simulink model "automata_learning"  (R2022a)
settings: Solver=FixedStepAuto  StartTime=0.0  StopTime=10.0  FixedStep=0.01  RelTol=1e-3
settings Model: Creator=diego  LastModifiedBy=diego

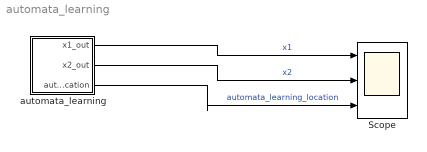
== system automata_learning ==
  Scope : Scope  NumInputPorts=3
  automata_learning : Stateflow chart  TreatAsAtomicUnit=on
  wires:
  automata_learning/1(x1_out) -> Scope/1  "x1"
  automata_learning/2(x2_out) -> Scope/2  "x2"
  automata_learning/3(automata_learning_location) -> Scope/3  "automata_learning_location"

== stateflow chart automata_learning/automata_learning ==
  settings: updateMethod=CONTINUOUS
  state loc1
    du:
    x1_dot = 0.153649240732193 * (exp(0.62066251039505 * x1 + 0.017139941453933716 * x2 + 0.2983952462673187) - 1.0) / (exp(0.62066251039505 * x1 + 0.017139941453933716 * x2 + 0.2983952462673187) + 1.0) - 0.2748902142047882 * (exp(0.430800199508667 * x1 + 0.22947368025779724 * x2 - 0.22418212890625) - 1.0) / (exp(0.430800199508667 * x1 + 0.22947368025779724 * x2 - 0.22418212890625) + 1.0) + 0.32443326711654663 * (exp(0.6266034245491028 * x2 - 0.5493556261062622 * x1 + 0.17436186969280243) - 1.0) / (exp(0.6266034245491028 * x2 - 0.5493556261062622 * x1 + 0.17436186969280243) + 1.0) + 0.3301161229610443 * (exp(0.6688907146453857 * x1 + 0.6354950666427612 * x2 + 0.28973063826560974) - 1.0) / (exp(0.6688907146453857 * x1 + 0.6354950666427612 * x2 + 0.28973063826560974) + 1.0) + 0.3717308044433594 * (exp(0.5966212749481201 * x1 - 0.30495092272758484 * x2 + 0.17112641036510468) - 1.0) / (exp(0.5966212749481201 * x1 - 0.30495092272758484 * x2 + 0.17112641036510468) + 1.0) + 0.15974511206150055 * (exp(0.5138949155807495 * x2 - 0.872249186038971 * x1 + 0.12989071011543274) - 1.0) / (exp(0.5138949155807495 * x2 - 0.872249186038971 * x1 + 0.12989071011543274) + 1.0) + 0.09516903012990952 * (exp(0.5174744129180908 * x1 - 0.458869606256485 * x2 + 0.07007770240306854) - 1.0) / (exp(0.5174744129180908 * x1 - 0.458869606256485 * x2 + 0.07007770240306854) + 1.0) + 0.13788394629955292 * (exp(0.3413529098033905 * x1 - 0.13695278763771057 * x2 + 0.0960288867354393) - 1.0) / (exp(0.3413529098033905 * x1 - 0.13695278763771057 * x2 + 0.0960288867354393) + 1.0) + 0.23488743603229523 * (exp(0.459713339805603 * x1 + 0.2586129903793335 * x2 + 0.14161019027233124) - 1.0) / (exp(0.459713339805603 * x1 + 0.2586129903793335 * x2 + 0.14161019027233124) + 1.0) - 0.38932523131370544 * (exp(0.16752173006534576 * x1 + 0.30755898356437683 * x2 - 0.18332701921463013) - 1.0) / (exp(0.16752173006534576 * x1 + 0.30755898356437683 * x2 - 0.18332701921463013) + 1.0) + 0.4114132523536682 * (exp(0.4421512186527252 * x2 - 0.0019959965720772743 * x1 + 0.1608879119157791) - 1.0) / (exp(0.4421512186527252 * x2 - 0.0019959965720772743 * x1 + 0.1608879119157791) + 1.0) + 0.2618536949157715 * (exp(0.7581536173820496 * x2 - 0.5491491556167603 * x1 + 0.1869184970855713) - 1.0) / (exp(0.7581536173820496 * x2 - 0.5491491556167603 * x1 + 0.1869184970855713) + 1.0) - 0.28562095761299133 * (exp(0.5797051787376404 * x1 + 0.4280661344528198 * x2 - 0.32014745473861694) - 1.0) / (exp(0.5797051787376404 * x1 + 0.4280661344528198 * x2 - 0.32014745473861694) + 1.0) - 0.022995460778474808 * (exp(0.5465248227119446 * x1 - 0.7955937385559082 * x2 + 0.025239817798137665) - 1.0) / (exp(0.5465248227119446 * x1 - 0.7955937385559082 * x2 + 0.025239817798137665) + 1.0) + 0.40521523356437683 * (exp(0.015660669654607773 * x1 - 0.0256962887942791 * x2 + 0.21741506457328796) - 1.0) / (exp(0.015660669654607773 * x1 - 0.0256962887942791 * x2 + 0.21741506457328796) + 1.0) + 0.35603979229927063 * (exp(0.20083804428577423 * x1 - 0.17433811724185944 * x2 + 0.1748630851507187) - 1.0) / (exp(0.20083804428577423 * x1 - 0.17433811724185944 * x2 + 0.1748630851507187) + 1.0) + 0.36211273074150085 * (exp(0.09791313111782074 * x1 + 0.12835988402366638 * x2 + 0.23166249692440033) - 1.0) / (exp(0.09791313111782074 * x1 + 0.12835988402366638 * x2 + 0.23166249692440033) + 1.0) + 0.05281674489378929 * (exp(0.6614029407501221 * x1 - 0.7321106195449829 * x2 + 0.10560699552297592) - 1.0) / (exp(0.6614029407501221 * x1 - 0.7321106195449829 * x2 + 0.10560699552297592) + 1.0) + 0.2983291745185852 * (exp(0.6240413188934326 * x2 - 0.6195738315582275 * x1 + 0.24919748306274414) - 1.0) / (exp(0.6240413188934326 * x2 - 0.6195738315582275 * x1 + 0.24919748306274414) + 1.0) - 0.07643954455852509 * (exp(0.37432658672332764 * x1 + 0.13084420561790466 * x2 - 0.061473298817873) - 1.0) / (exp(0.37432658672332764 * x1 + 0.13084420561790466 * x2 - 0.061473298817873) + 1.0) + 0.07931482791900635 * (exp(0.6290643215179443 * x1 + 0.7032239437103271 * x2 + 0.029886124655604362) - 1.0) / (exp(0.6290643215179443 * x1 + 0.7032239437103271 * x2 + 0.029886124655604362) + 1.0) + 0.3452206552028656 * (exp(0.46229633688926697 * x1 - 0.17825168371200562 * x2 + 0.33221080899238586) - 1.0) / (exp(0.46229633688926697 * x1 - 0.17825168371200562 * x2 + 0.33221080899238586) + 1.0) - 0.3357248306274414 * (exp(0.32255837321281433 * x1 + 0.4906807243824005 * x2 - 0.171269491314888) - 1.0) / (exp(0.32255837321281433 * x1 + 0.4906807243824005 * x2 - 0.171269491314888) + 1.0) + 0.032010987401008606 * (exp(0.49095281958580017 * x1 - 0.07064257562160492 * x2 + 0.20939995348453522) - 1.0) / (exp(0.49095281958580017 * x1 - 0.07064257562160492 * x2 + 0.20939995348453522) + 1.0) + 0.26413223147392273 * (exp(0.45438820123672485 * x1 - 0.2572150230407715 * x2 + 0.24137400090694427) - 1.0) / (exp(0.45438820123672485 * x1 - 0.2572150230407715 * x2 + 0.24137400090694427) + 1.0) - 0.3747853934764862 * (exp(0.8867902755737305 * x1 + 0.4323332607746124 * x2 - 0.3189244270324707) - 1.0) / (exp(0.8867902755737305 * x1 + 0.4323332607746124 * x2 - 0.3189244270324707) + 1.0) + 0.41086137294769287 * (exp(0.36686065793037415 * x2 - 0.000020963780116289854 * x1 + 0.24850977957248688) - 1.0) / (exp(0.36686065793037415 * x2 - 0.000020963780116289854 * x1 + 0.24850977957248688) + 1.0) + 0.5473085641860962 * (exp(0.20481422543525696 * x1 - 0.47845104336738586 * x2 + 0.3234947621822357) - 1.0) / (exp(0.20481422543525696 * x1 - 0.47845104336738586 * x2 + 0.3234947621822357) + 1.0) + 0.05670561641454697 * (exp(0.34265992045402527 * x1 + 0.7918558120727539 * x2 + 0.11939319968223572) - 1.0) / (exp(0.34265992045402527 * x1 + 0.7918558120727539 * x2 + 0.11939319968223572) + 1.0) + 0.39071744680404663 * (exp(0.49077701568603516 * x1 - 0.11882556974887848 * x2 + 0.2540743947029114) - 1.0) / (exp(0.49077701568603516 * x1 - 0.11882556974887848 * x2 + 0.2540743947029114) + 1.0) + 0.13067974150180817;
    x2_dot = 0.4149567782878876 * (exp(0.430800199508667 * x1 + 0.22947368025779724 * x2 - 0.22418212890625) - 1.0) / (exp(0.430800199508667 * x1 + 0.22947368025779724 * x2 - 0.22418212890625) + 1.0) + 0.033265016973018646 * (exp(0.62066251039505 * x1 + 0.017139941453933716 * x2 + 0.2983952462673187) - 1.0) / (exp(0.62066251039505 * x1 + 0.017139941453933716 * x2 + 0.2983952462673187) + 1.0) + 0.11906763911247253 * (exp(0.6266034245491028 * x2 - 0.5493556261062622 * x1 + 0.17436186969280243) - 1.0) / (exp(0.6266034245491028 * x2 - 0.5493556261062622 * x1 + 0.17436186969280243) + 1.0) + 0.09495125710964203 * (exp(0.6688907146453857 * x1 + 0.6354950666427612 * x2 + 0.28973063826560974) - 1.0) / (exp(0.6688907146453857 * x1 + 0.6354950666427612 * x2 + 0.28973063826560974) + 1.0) + 0.4443686902523041 * (exp(0.5966212749481201 * x1 - 0.30495092272758484 * x2 + 0.17112641036510468) - 1.0) / (exp(0.5966212749481201 * x1 - 0.30495092272758484 * x2 + 0.17112641036510468) + 1.0) - 0.4195578992366791 * (exp(0.5138949155807495 * x2 - 0.872249186038971 * x1 + 0.12989071011543274) - 1.0) / (exp(0.5138949155807495 * x2 - 0.872249186038971 * x1 + 0.12989071011543274) + 1.0) + 0.46499332785606384 * (exp(0.5174744129180908 * x1 - 0.458869606256485 * x2 + 0.07007770240306854) - 1.0) / (exp(0.5174744129180908 * x1 - 0.458869606256485 * x2 + 0.07007770240306854) + 1.0) + 0.3947281837463379 * (exp(0.3413529098033905 * x1 - 0.13695278763771057 * x2 + 0.0960288867354393) - 1.0) / (exp(0.3413529098033905 * x1 - 0.13695278763771057 * x2 + 0.0960288867354393) + 1.0) + 0.36730241775512695 * (exp(0.459713339805603 * x1 + 0.2586129903793335 * x2 + 0.14161019027233124) - 1.0) / (exp(0.459713339805603 * x1 + 0.2586129903793335 * x2 + 0.14161019027233124) + 1.0) - 0.266009658575058 * (exp(0.16752173006534576 * x1 + 0.30755898356437683 * x2 - 0.18332701921463013) - 1.0) / (exp(0.16752173006534576 * x1 + 0.30755898356437683 * x2 - 0.18332701921463013) + 1.0) + 0.4192095696926117 * (exp(0.4421512186527252 * x2 - 0.0019959965720772743 * x1 + 0.1608879119157791) - 1.0) / (exp(0.4421512186527252 * x2 - 0.0019959965720772743 * x1 + 0.1608879119157791) + 1.0) + 0.008743703365325928 * (exp(0.7581536173820496 * x2 - 0.5491491556167603 * x1 + 0.1869184970855713) - 1.0) / (exp(0.7581536173820496 * x2 - 0.5491491556167603 * x1 + 0.1869184970855713) + 1.0) + 0.14651131629943848 * (exp(0.5797051787376404 * x1 + 0.4280661344528198 * x2 - 0.32014745473861694) - 1.0) / (exp(0.5797051787376404 * x1 + 0.4280661344528198 * x2 - 0.32014745473861694) + 1.0) - 0.3324713110923767 * (exp(0.5465248227119446 * x1 - 0.7955937385559082 * x2 + 0.025239817798137665) - 1.0) / (exp(0.5465248227119446 * x1 - 0.7955937385559082 * x2 + 0.025239817798137665) + 1.0) + 0.1831395924091339 * (exp(0.015660669654607773 * x1 - 0.0256962887942791 * x2 + 0.21741506457328796) - 1.0) / (exp(0.015660669654607773 * x1 - 0.0256962887942791 * x2 + 0.21741506457328796) + 1.0) + 0.3701251149177551 * (exp(0.20083804428577423 * x1 - 0.17433811724185944 * x2 + 0.1748630851507187) - 1.0) / (exp(0.20083804428577423 * x1 - 0.17433811724185944 * x2 + 0.1748630851507187) + 1.0) + 0.1405045986175537 * (exp(0.09791313111782074 * x1 + 0.12835988402366638 * x2 + 0.23166249692440033) - 1.0) / (exp(0.09791313111782074 * x1 + 0.12835988402366638 * x2 + 0.23166249692440033) + 1.0) - 0.22994273900985718 * (exp(0.6614029407501221 * x1 - 0.7321106195449829 * x2 + 0.10560699552297592) - 1.0) / (exp(0.6614029407501221 * x1 - 0.7321106195449829 * x2 + 0.10560699552297592) + 1.0) - 0.3847588896751404 * (exp(0.6240413188934326 * x2 - 0.6195738315582275 * x1 + 0.24919748306274414) - 1.0) / (exp(0.6240413188934326 * x2 - 0.6195738315582275 * x1 + 0.24919748306274414) + 1.0) + 0.43302276730537415 * (exp(0.37432658672332764 * x1 + 0.13084420561790466 * x2 - 0.061473298817873) - 1.0) / (exp(0.37432658672332764 * x1 + 0.13084420561790466 * x2 - 0.061473298817873) + 1.0) + 0.3945055603981018 * (exp(0.6290643215179443 * x1 + 0.7032239437103271 * x2 + 0.029886124655604362) - 1.0) / (exp(0.6290643215179443 * x1 + 0.7032239437103271 * x2 + 0.029886124655604362) + 1.0) - 0.23404325544834137 * (exp(0.46229633688926697 * x1 - 0.17825168371200562 * x2 + 0.33221080899238586) - 1.0) / (exp(0.46229633688926697 * x1 - 0.17825168371200562 * x2 + 0.33221080899238586) + 1.0) - 0.26820316910743713 * (exp(0.32255837321281433 * x1 + 0.4906807243824005 * x2 - 0.171269491314888) - 1.0) / (exp(0.32255837321281433 * x1 + 0.4906807243824005 * x2 - 0.171269491314888) + 1.0) + 0.058586183935403824 * (exp(0.49095281958580017 * x1 - 0.07064257562160492 * x2 + 0.20939995348453522) - 1.0) / (exp(0.49095281958580017 * x1 - 0.07064257562160492 * x2 + 0.20939995348453522) + 1.0) + 0.1390489935874939 * (exp(0.45438820123672485 * x1 - 0.2572150230407715 * x2 + 0.24137400090694427) - 1.0) / (exp(0.45438820123672485 * x1 - 0.2572150230407715 * x2 + 0.24137400090694427) + 1.0) + 0.4438546895980835 * (exp(0.8867902755737305 * x1 + 0.4323332607746124 * x2 - 0.3189244270324707) - 1.0) / (exp(0.8867902755737305 * x1 + 0.4323332607746124 * x2 - 0.3189244270324707) + 1.0) + 0.0753171443939209 * (exp(0.36686065793037415 * x2 - 0.000020963780116289854 * x1 + 0.24850977957248688) - 1.0) / (exp(0.36686065793037415 * x2 - 0.000020963780116289854 * x1 + 0.24850977957248688) + 1.0) - 0.1991405040025711 * (exp(0.20481422543525696 * x1 - 0.47845104336738586 * x2 + 0.3234947621822357) - 1.0) / (exp(0.20481422543525696 * x1 - 0.47845104336738586 * x2 + 0.3234947621822357) + 1.0) - 0.3242756724357605 * (exp(0.34265992045402527 * x1 + 0.7918558120727539 * x2 + 0.11939319968223572) - 1.0) / (exp(0.34265992045402527 * x1 + 0.7918558120727539 * x2 + 0.11939319968223572) + 1.0) + 0.1375180333852768 * (exp(0.49077701568603516 * x1 - 0.11882556974887848 * x2 + 0.2540743947029114) - 1.0) / (exp(0.49077701568603516 * x1 - 0.11882556974887848 * x2 + 0.2540743947029114) + 1.0) - 0.002385741099715233;
    x1_out=x1;
    x2_out=x2;
    automata_learning_location =1;
  state loc2
    du:
    x1_dot = 0.12665143609046936 * (exp(0.521274983882904 * x2 - 0.15485931932926178 * x1 + 0.12516500055789948) - 1.0) / (exp(0.521274983882904 * x2 - 0.15485931932926178 * x1 + 0.12516500055789948) + 1.0) - 0.03703930601477623 * (exp(0.3801111578941345 * x1 + 0.4741904139518738 * x2 - 0.2445288449525833) - 1.0) / (exp(0.3801111578941345 * x1 + 0.4741904139518738 * x2 - 0.2445288449525833) + 1.0) + 0.6335803866386414 * (exp(0.4992769956588745 * x1 - 0.7368530631065369 * x2 + 0.2410757690668106) - 1.0) / (exp(0.4992769956588745 * x1 - 0.7368530631065369 * x2 + 0.2410757690668106) + 1.0) + 0.043215252459049225 * (exp(0.01397448405623436 * x1 - 0.4834722578525543 * x2 + 0.21923306584358215) - 1.0) / (exp(0.01397448405623436 * x1 - 0.4834722578525543 * x2 + 0.21923306584358215) + 1.0) + 0.2113444060087204 * (exp(0.5212129354476929 * x1 - 0.36429619789123535 * x2 + 0.27187180519104004) - 1.0) / (exp(0.5212129354476929 * x1 - 0.36429619789123535 * x2 + 0.27187180519104004) + 1.0) - 0.3356776535511017 * (exp(0.6180296540260315 * x1 + 0.3545454442501068 * x2 + 0.12871329486370087) - 1.0) / (exp(0.6180296540260315 * x1 + 0.3545454442501068 * x2 + 0.12871329486370087) + 1.0) - 0.10880768299102783 * (exp(0.5730214715003967 * x1 - 0.2724354565143585 * x2 + 0.20432481169700623) - 1.0) / (exp(0.5730214715003967 * x1 - 0.2724354565143585 * x2 + 0.20432481169700623) + 1.0) - 0.12154649198055267 * (exp(0.23054413497447968 * x1 - 0.5182762742042542 * x2 + 0.1265276074409485) - 1.0) / (exp(0.23054413497447968 * x1 - 0.5182762742042542 * x2 + 0.1265276074409485) + 1.0) - 0.14984062314033508 * (exp(0.30335184931755066 * x1 + 0.2244175374507904 * x2 + 0.25061026215553284) - 1.0) / (exp(0.30335184931755066 * x1 + 0.2244175374507904 * x2 + 0.25061026215553284) + 1.0) - 0.40790629386901855 * (exp(0.21870259940624237 * x1 + 0.5387592911720276 * x2 + 0.03809625282883644) - 1.0) / (exp(0.21870259940624237 * x1 + 0.5387592911720276 * x2 + 0.03809625282883644) + 1.0) - 0.15038713812828064 * (exp(0.19810104370117188 * x1 - 0.12814362347126007 * x2 + 0.18356406688690186) - 1.0) / (exp(0.19810104370117188 * x1 - 0.12814362347126007 * x2 + 0.18356406688690186) + 1.0) - 0.19513456523418427 * (exp(0.7527180910110474 * x1 + 0.36526915431022644 * x2 - 0.2935789227485657) - 1.0) / (exp(0.7527180910110474 * x1 + 0.36526915431022644 * x2 - 0.2935789227485657) + 1.0) - 0.42879360914230347 * (exp(0.5669860243797302 * x1 + 0.565645158290863 * x2 + 0.12304074317216873) - 1.0) / (exp(0.5669860243797302 * x1 + 0.565645158290863 * x2 + 0.12304074317216873) + 1.0) + 0.13006073236465454 * (exp(0.12214836478233337 * x2 - 0.543998658657074 * x1 + 0.15256726741790771) - 1.0) / (exp(0.12214836478233337 * x2 - 0.543998658657074 * x1 + 0.15256726741790771) + 1.0) + 0.14575129747390747 * (exp(0.6980375647544861 * x1 + 0.33853843808174133 * x2 + 0.3808814585208893) - 1.0) / (exp(0.6980375647544861 * x1 + 0.33853843808174133 * x2 + 0.3808814585208893) + 1.0) + 0.09190955758094788 * (exp(0.3255921006202698 * x2 - 0.20148040354251862 * x1 + 0.35358673334121704) - 1.0) / (exp(0.3255921006202698 * x2 - 0.20148040354251862 * x1 + 0.35358673334121704) + 1.0) - 0.5171889066696167 * (exp(0.6075751185417175 * x1 + 0.41354966163635254 * x2 + 0.18314096331596375) - 1.0) / (exp(0.6075751185417175 * x1 + 0.41354966163635254 * x2 + 0.18314096331596375) + 1.0) - 0.14301341772079468 * (exp(0.7139869928359985 * x2 - 0.45711761713027954 * x1 + 0.2765464782714844) - 1.0) / (exp(0.7139869928359985 * x2 - 0.45711761713027954 * x1 + 0.2765464782714844) + 1.0) - 0.06974461674690247 * (exp(0.7396500706672668 * x1 + 0.05845750495791435 * x2 + 0.2551769018173218) - 1.0) / (exp(0.7396500706672668 * x1 + 0.05845750495791435 * x2 + 0.2551769018173218) + 1.0) - 0.03698032349348068 * (exp(0.2508452832698822 * x2 - 0.7632717490196228 * x1 + 0.2401130050420761) - 1.0) / (exp(0.2508452832698822 * x2 - 0.7632717490196228 * x1 + 0.2401130050420761) + 1.0) - 0.3060373365879059 * (exp(0.025464177131652832 * x1 + 0.2838376462459564 * x2 + 0.21075984835624695) - 1.0) / (exp(0.025464177131652832 * x1 + 0.2838376462459564 * x2 + 0.21075984835624695) + 1.0) - 0.034435901790857315 * (exp(0.7091931104660034 * x1 + 0.5794293284416199 * x2 - 0.23994916677474976) - 1.0) / (exp(0.7091931104660034 * x1 + 0.5794293284416199 * x2 - 0.23994916677474976) + 1.0) - 0.2008693516254425 * (exp(0.22183528542518616 * x1 + 0.7863845229148865 * x2 + 0.15160590410232544) - 1.0) / (exp(0.22183528542518616 * x1 + 0.7863845229148865 * x2 + 0.15160590410232544) + 1.0) - 0.42737627029418945 * (exp(0.040710680186748505 * x1 + 0.8926408886909485 * x2 - 0.38132381439208984) - 1.0) / (exp(0.040710680186748505 * x1 + 0.8926408886909485 * x2 - 0.38132381439208984) + 1.0) - 0.46405455470085144 * (exp(0.7100028991699219 * x2 - 0.48056063055992126 * x1 + 0.16554595530033112) - 1.0) / (exp(0.7100028991699219 * x2 - 0.48056063055992126 * x1 + 0.16554595530033112) + 1.0) - 0.034204356372356415 * (exp(0.7528899908065796 * x1 + 0.5968327522277832 * x2 - 0.2467477172613144) - 1.0) / (exp(0.7528899908065796 * x1 + 0.5968327522277832 * x2 - 0.2467477172613144) + 1.0) + 0.18453453481197357 * (exp(0.3175884783267975 * x2 - 0.4910913109779358 * x1 + 0.19048462808132172) - 1.0) / (exp(0.3175884783267975 * x2 - 0.4910913109779358 * x1 + 0.19048462808132172) + 1.0) + 0.3044191598892212 * (exp(0.029053879901766777 * x1 - 0.427410751581192 * x2 + 0.3036733865737915) - 1.0) / (exp(0.029053879901766777 * x1 - 0.427410751581192 * x2 + 0.3036733865737915) + 1.0) - 0.1919207125902176 * (exp(0.574486255645752 * x1 + 0.24281814694404602 * x2 + 0.24069303274154663) - 1.0) / (exp(0.574486255645752 * x1 + 0.24281814694404602 * x2 + 0.24069303274154663) + 1.0) - 0.1355563849210739 * (exp(0.4902433454990387 * x1 - 0.4684576690196991 * x2 + 0.16988161206245422) - 1.0) / (exp(0.4902433454990387 * x1 - 0.4684576690196991 * x2 + 0.16988161206245422) + 1.0) - 0.0604635626077652;
    x2_dot = 0.29203087091445923 * (exp(0.3801111578941345 * x1 + 0.4741904139518738 * x2 - 0.2445288449525833) - 1.0) / (exp(0.3801111578941345 * x1 + 0.4741904139518738 * x2 - 0.2445288449525833) + 1.0) - 0.18211862444877625 * (exp(0.521274983882904 * x2 - 0.15485931932926178 * x1 + 0.12516500055789948) - 1.0) / (exp(0.521274983882904 * x2 - 0.15485931932926178 * x1 + 0.12516500055789948) + 1.0) - 0.27369001507759094 * (exp(0.4992769956588745 * x1 - 0.7368530631065369 * x2 + 0.2410757690668106) - 1.0) / (exp(0.4992769956588745 * x1 - 0.7368530631065369 * x2 + 0.2410757690668106) + 1.0) - 0.13422976434230804 * (exp(0.01397448405623436 * x1 - 0.4834722578525543 * x2 + 0.21923306584358215) - 1.0) / (exp(0.01397448405623436 * x1 - 0.4834722578525543 * x2 + 0.21923306584358215) + 1.0) - 0.26479941606521606 * (exp(0.5212129354476929 * x1 - 0.36429619789123535 * x2 + 0.27187180519104004) - 1.0) / (exp(0.5212129354476929 * x1 - 0.36429619789123535 * x2 + 0.27187180519104004) + 1.0) - 0.07722172886133194 * (exp(0.6180296540260315 * x1 + 0.3545454442501068 * x2 + 0.12871329486370087) - 1.0) / (exp(0.6180296540260315 * x1 + 0.3545454442501068 * x2 + 0.12871329486370087) + 1.0) - 0.28563281893730164 * (exp(0.5730214715003967 * x1 - 0.2724354565143585 * x2 + 0.20432481169700623) - 1.0) / (exp(0.5730214715003967 * x1 - 0.2724354565143585 * x2 + 0.20432481169700623) + 1.0) - 0.009569618850946426 * (exp(0.23054413497447968 * x1 - 0.5182762742042542 * x2 + 0.1265276074409485) - 1.0) / (exp(0.23054413497447968 * x1 - 0.5182762742042542 * x2 + 0.1265276074409485) + 1.0) - 0.287971168756485 * (exp(0.30335184931755066 * x1 + 0.2244175374507904 * x2 + 0.25061026215553284) - 1.0) / (exp(0.30335184931755066 * x1 + 0.2244175374507904 * x2 + 0.25061026215553284) + 1.0) + 0.020914098247885704 * (exp(0.21870259940624237 * x1 + 0.5387592911720276 * x2 + 0.03809625282883644) - 1.0) / (exp(0.21870259940624237 * x1 + 0.5387592911720276 * x2 + 0.03809625282883644) + 1.0) - 0.17691387236118317 * (exp(0.19810104370117188 * x1 - 0.12814362347126007 * x2 + 0.18356406688690186) - 1.0) / (exp(0.19810104370117188 * x1 - 0.12814362347126007 * x2 + 0.18356406688690186) + 1.0) + 0.3997935652732849 * (exp(0.7527180910110474 * x1 + 0.36526915431022644 * x2 - 0.2935789227485657) - 1.0) / (exp(0.7527180910110474 * x1 + 0.36526915431022644 * x2 - 0.2935789227485657) + 1.0) - 0.14379826188087463 * (exp(0.5669860243797302 * x1 + 0.565645158290863 * x2 + 0.12304074317216873) - 1.0) / (exp(0.5669860243797302 * x1 + 0.565645158290863 * x2 + 0.12304074317216873) + 1.0) - 0.24429135024547577 * (exp(0.12214836478233337 * x2 - 0.543998658657074 * x1 + 0.15256726741790771) - 1.0) / (exp(0.12214836478233337 * x2 - 0.543998658657074 * x1 + 0.15256726741790771) + 1.0) - 0.39709171652793884 * (exp(0.6980375647544861 * x1 + 0.33853843808174133 * x2 + 0.3808814585208893) - 1.0) / (exp(0.6980375647544861 * x1 + 0.33853843808174133 * x2 + 0.3808814585208893) + 1.0) - 0.47019162774086 * (exp(0.3255921006202698 * x2 - 0.20148040354251862 * x1 + 0.35358673334121704) - 1.0) / (exp(0.3255921006202698 * x2 - 0.20148040354251862 * x1 + 0.35358673334121704) + 1.0) - 0.428403377532959 * (exp(0.6075751185417175 * x1 + 0.41354966163635254 * x2 + 0.18314096331596375) - 1.0) / (exp(0.6075751185417175 * x1 + 0.41354966163635254 * x2 + 0.18314096331596375) + 1.0) - 0.23058690130710602 * (exp(0.7139869928359985 * x2 - 0.45711761713027954 * x1 + 0.2765464782714844) - 1.0) / (exp(0.7139869928359985 * x2 - 0.45711761713027954 * x1 + 0.2765464782714844) + 1.0) - 0.12516361474990845 * (exp(0.7396500706672668 * x1 + 0.05845750495791435 * x2 + 0.2551769018173218) - 1.0) / (exp(0.7396500706672668 * x1 + 0.05845750495791435 * x2 + 0.2551769018173218) + 1.0) - 0.24258922040462494 * (exp(0.2508452832698822 * x2 - 0.7632717490196228 * x1 + 0.2401130050420761) - 1.0) / (exp(0.2508452832698822 * x2 - 0.7632717490196228 * x1 + 0.2401130050420761) + 1.0) - 0.26785042881965637 * (exp(0.025464177131652832 * x1 + 0.2838376462459564 * x2 + 0.21075984835624695) - 1.0) / (exp(0.025464177131652832 * x1 + 0.2838376462459564 * x2 + 0.21075984835624695) + 1.0) + 0.19651581346988678 * (exp(0.7091931104660034 * x1 + 0.5794293284416199 * x2 - 0.23994916677474976) - 1.0) / (exp(0.7091931104660034 * x1 + 0.5794293284416199 * x2 - 0.23994916677474976) + 1.0) - 0.10432932525873184 * (exp(0.22183528542518616 * x1 + 0.7863845229148865 * x2 + 0.15160590410232544) - 1.0) / (exp(0.22183528542518616 * x1 + 0.7863845229148865 * x2 + 0.15160590410232544) + 1.0) + 0.2659221887588501 * (exp(0.040710680186748505 * x1 + 0.8926408886909485 * x2 - 0.38132381439208984) - 1.0) / (exp(0.040710680186748505 * x1 + 0.8926408886909485 * x2 - 0.38132381439208984) + 1.0) - 0.2799898386001587 * (exp(0.7100028991699219 * x2 - 0.48056063055992126 * x1 + 0.16554595530033112) - 1.0) / (exp(0.7100028991699219 * x2 - 0.48056063055992126 * x1 + 0.16554595530033112) + 1.0) + 0.24723581969738007 * (exp(0.7528899908065796 * x1 + 0.5968327522277832 * x2 - 0.2467477172613144) - 1.0) / (exp(0.7528899908065796 * x1 + 0.5968327522277832 * x2 - 0.2467477172613144) + 1.0) - 0.31184446811676025 * (exp(0.3175884783267975 * x2 - 0.4910913109779358 * x1 + 0.19048462808132172) - 1.0) / (exp(0.3175884783267975 * x2 - 0.4910913109779358 * x1 + 0.19048462808132172) + 1.0) - 0.32754766941070557 * (exp(0.029053879901766777 * x1 - 0.427410751581192 * x2 + 0.3036733865737915) - 1.0) / (exp(0.029053879901766777 * x1 - 0.427410751581192 * x2 + 0.3036733865737915) + 1.0) - 0.4281812310218811 * (exp(0.574486255645752 * x1 + 0.24281814694404602 * x2 + 0.24069303274154663) - 1.0) / (exp(0.574486255645752 * x1 + 0.24281814694404602 * x2 + 0.24069303274154663) + 1.0) - 0.10796092450618744 * (exp(0.4902433454990387 * x1 - 0.4684576690196991 * x2 + 0.16988161206245422) - 1.0) / (exp(0.4902433454990387 * x1 - 0.4684576690196991 * x2 + 0.16988161206245422) + 1.0) - 0.12882886826992035;
    x1_out=x1;
    x2_out=x2;
    automata_learning_location =2;
  loc1 -> loc2 : [0.0009391 * x2 - 0.4996 * x1 + 1.0 < 0.0]
  (default) -> loc1 : {x1 = 0.0;
      | x2 = 0.0;}
  loc2 -> loc1 : [0.01034 * x1 + 196.7 * x2 + 1.0 < 0.0]
  data: x1_out output; x1 local; x2_out output; x2 local; automata_learning_location output
  data x1 settings: updateMethod=SF_CONTINUOUS_TIME_DATA
  data x2 settings: updateMethod=SF_CONTINUOUS_TIME_DATA
